simulink model "untitled"  (R2020b)
settings: Solver=VariableStepAuto  StartTime=0.0  StopTime=200.0  RelTol=1e-3
libraries: simulink x1
settings Model: Creator=morro  LastModifiedBy=morro

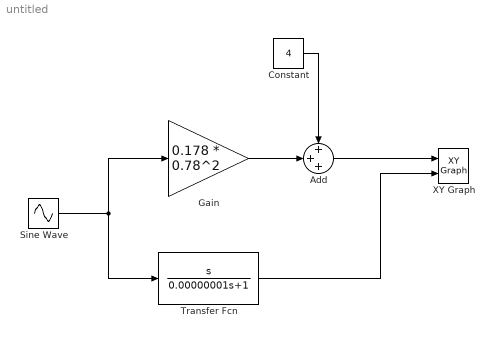
== system untitled ==
  Add : Sum  Inputs=+++
  Constant : Constant  Value=4
  Gain : Gain  Gain=0.178 * 0.78^2
  Sine Wave : Sin  Amplitude=200  Frequency=0.78  SampleTime=0
  Transfer Fcn : TransferFcn  Numerator=[1 0]  Denominator=[0.00000001 1]
  XY Graph : simulink/Sinks/XY Graph  xmin=-25  xmax=25  ymin=-200  ymax=200  st=-1
  wires:
  Sine Wave/1 -> Gain/1, Transfer Fcn/1
  Gain/1 -> Add/2
  Constant/1 -> Add/1
  Add/1 -> XY Graph/1
  Transfer Fcn/1 -> XY Graph/2
